simulink model "uz_drive_model"  (R2021b)
settings: Solver=FixedStepAuto  StartTime=0.0  StopTime=0.6  RelTol=1e-3
PreLoadFcn:
  | uz_pmsm_model_9ph_init_parameter
values from neighbouring files (symbols this model uses):
  c = 2/9*cat(1,tl1,tl2,tl3,tl4,tl5,tl6,tl7,tl8,tl9)    [uz_pmsm_model_9ph_init_parameter.m]
  f_pwm = 50000    [uz_pmsm_model_9ph_init_parameter.m]
  friction_coefficient = 0.001    [uz_pmsm_model_9ph_init_parameter.m]
  inertia = 0.001    [uz_pmsm_model_9ph_init_parameter.m]
  k_i_d = R_1/(2*tau_sum)    (= 78250)    [uz_pmsm_model_9ph_init_parameter.m]
  k_i_q = R_1/(2*tau_sum)    (= 78250)    [uz_pmsm_model_9ph_init_parameter.m]
  k_p_d = L_d/(2*tau_sum)    (= 1250)    [uz_pmsm_model_9ph_init_parameter.m]
  k_p_q = L_q/(2*tau_sum)    (= 1250)    [uz_pmsm_model_9ph_init_parameter.m]
  L_d = 0.5    [uz_pmsm_model_9ph_init_parameter.m]
  L_o1 = Lls    (= 0.08)    [uz_pmsm_model_9ph_init_parameter.m]
  L_o2 = Lls    (= 0.08)    [uz_pmsm_model_9ph_init_parameter.m]
  L_q = 0.5    [uz_pmsm_model_9ph_init_parameter.m]
  L_x1 = Lls    (= 0.08)    [uz_pmsm_model_9ph_init_parameter.m]
  L_x2 = Lls    (= 0.08)    [uz_pmsm_model_9ph_init_parameter.m]
  L_y1 = Lls    (= 0.08)    [uz_pmsm_model_9ph_init_parameter.m]
  L_y2 = Lls    (= 0.08)    [uz_pmsm_model_9ph_init_parameter.m]
  L_zero = Lls    (= 0.08)    [uz_pmsm_model_9ph_init_parameter.m]
  lim_pi = udc/2    (= 280)    [uz_pmsm_model_9ph_init_parameter.m]
  polepair = 2    [uz_pmsm_model_9ph_init_parameter.m]
  psi_pm = 0.6    [uz_pmsm_model_9ph_init_parameter.m]
  R_1 = 31.3    [uz_pmsm_model_9ph_init_parameter.m]
  static_friction_torque = 0.001    [uz_pmsm_model_9ph_init_parameter.m]
  ts = 2/1e6    (= 2e-06)    [uz_pmsm_model_9ph_init_parameter.m]
  udc = 560    [uz_pmsm_model_9ph_init_parameter.m]
undefined symbols (not defined in the file or in its folder): Kpd, Tnd
libraries: nesl_utility x51, fl_lib x43, ee_lib x27, eePwmGeneratorMultilevel x9, simulink x2, slpidlib x2, spsAlphaBetaZerotodq0Lib x1, pid_lib x1, spsdq0toAlphaBetaZeroLib x1
(part 4 of 4)

== system uz_drive_model/Subsystem4/uz_pmsm_model_9ph/pmsm/integrator7 ==
  in : Inport
  reset : Inport  Port=2
  Delay1 : Delay  DelayLength=1  ExternalReset=Level
      settings: InputPortMap=u0,r5
  Gain : Gain  Gain=ts  OutDataTypeStr=Inherit: Same as input
  Sum3 : Sum  Inputs=|++  OutDataTypeStr=Inherit: Same as first input
  outt : Outport
  wires:
  reset/1 -> Delay1/2
  Gain/1 -> Sum3/1
  in/1 -> Gain/1
  Delay1/1 -> outt/1, Sum3/2
  Sum3/1 -> Delay1/1

== system uz_drive_model/Subsystem4/uz_pmsm_model_9ph/pmsm/integrator8 ==
  in : Inport
  reset : Inport  Port=2
  Delay1 : Delay  DelayLength=1  ExternalReset=Level
      settings: InputPortMap=u0,r5
  Gain : Gain  Gain=ts  OutDataTypeStr=Inherit: Same as input
  Sum3 : Sum  Inputs=|++  OutDataTypeStr=Inherit: Same as first input
  outt : Outport
  wires:
  reset/1 -> Delay1/2
  Gain/1 -> Sum3/1
  in/1 -> Gain/1
  Delay1/1 -> outt/1, Sum3/2
  Sum3/1 -> Delay1/1
